simulink model "Simulador_Simulink"  (R2019b)
settings: Solver=FixedStepAuto  StartTime=0.0  StopTime=0.5  FixedStep=1e-6  RelTol=1e-3
model workspace (MAT data in the model file):
  SELDACA = 0
  SELPWM1A = 0
  SELPWM1B = 0
  SELPWM2A = 0
  SELPWM2B = 0
  SELPWM3A = 0
  SELPWM3B = 0
  Salidas_Reales = 0
values from neighbouring files (symbols this model uses):
  Dec = 1    [Sotfware_Matlab.m]
  Freq_Conmutacion = 10e3    (= 10000)    [Sotfware_Matlab.m]
  Ib = 2.5    [Sotfware_Matlab.m]
  Ireg_PI = tan((90 + Fc_pi)*pi/180)/wo_pi    [Sotfware_Matlab.m]
  Kreg_P = 1/AP    [Sotfware_Matlab.m]
  Kreg_PI = Ac_pi*Ireg_PI*wo_pi / sqrt(1 + (Ireg_PI*wo_pi)^2)    [Sotfware_Matlab.m]
  Lb = Zb/wb    [Sotfware_Matlab.m]
  Lpu = X_ind/ Lb    [Sotfware_Matlab.m]
  m = 0.5    [Sotfware_Matlab.m]
  Rpu = R_ind / Zb    [Sotfware_Matlab.m]
  T_pwm = 1/Freq_Conmutacion    (= 0.0001)    [Sotfware_Matlab.m]
  Ub = 0.61*Vdc / sqrt(3)    [Sotfware_Matlab.m]
  Vdc = 48    [Sotfware_Matlab.m]
  w1pu = 1    [Sotfware_Matlab.m]
  Zb = Ub/Ib    [Sotfware_Matlab.m]
libraries: powerlib x12, simulink x3, eeTransforms x3, electricdrivelib x1
settings Model: ParameterArgumentNames=SELDACA,SELPWM1A,SELPWM1B,SELPWM2A,SELPWM2B,SELPWM3A,SELPWM3B,Salidas_Reales  OrderedModelArguments=off  Creator=jorgesuarezporras  LastModifiedBy=jorge
settings SFSimCC: CustomCodeUndefinedFunction=UseInterfaceOnly

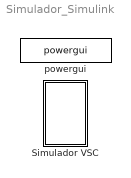
== system Simulador_Simulink ==
  Simulador VSC : Subsystem  mask{Parameter1A=Id, Parameter1B=Id Referencia, Parameter2A=Iq, Parameter2B=Iq Referencia, ParameterDAC=Ángulo transformada de Park, Parameter3A=Va, Parameter3B=Ia, Id_simulink=1, Iq_simulink=1, refd=Constante, refq=Constante, control=Control PI, K_proporcional=Kreg_P, b_proporcional=1, K_integral=Kreg_PI, I_integral=Ireg_PI, b_integral=1, tipolazo=Lazo Cerrado, mandod=0, mandoq=0, acoplamiento=on}
      mask prompts: Parameter1A "PWM1A"; Parameter1B "PWM1B"; Parameter2A "PWM2A"; Parameter2B "PWM2B"; ParameterDAC "DAC A"; Parameter3A "PWM3A"; Parameter3B "PWM3B"; Id_simulink "Id Referencia"; Iq_simulink "Iq Referencia"; refd "Forma de onda de referencia Id"; refq "Forma de onda de referencia Iq"; control "Selecciona el Control"; K_proporcional "K:"; b_proporcional "b:"; K_integral "K:"; I_integral "I:"; b_integral "b:"; tipolazo "Tipo de lazo"; mandod "Tensión de mando eje d  (md)"; mandoq "Tensión de mando eje q (mq)"
      mask init:
      | switch Parameter1A
      |     case 1
      |         SELPWM1A = 1;
      |     case 2
      |         SELPWM1A = 2;
      |     case 3
      |         SELPWM1A = 3;
      |     case 4
      |         SELPWM1A = 4;
      |     case 5
      |         SELPWM1A = 5;
      |     case 6
      |         SELPWM1A = 6;
      |     case 7
      |         SELPWM1A = 7;
      |     otherwise
      |         SELPWM1A = -1;
      | end
      | 
      | switch Parameter1B
      |     case 1
      |         SELPWM1B = 1;
      |     case 2
      |         SELPWM1B = 2;
      |     case 3
      |         SELPWM1B = 3;
      |     case 4
      |         SELPWM1B = 4;
      |     case 5
      |         SELPWM1B = 5;
      |     case 6
      |         SELPWM1B = 6;
      |     case 7
      |         SELPWM1B = 7;
      |     otherwise
      |         SELPWM1B = -1;
      | end
      | switch Parameter2A
      |     case 1
      |         SELPWM2A = 1;
      |     case 2
      |         SELPWM2A = 2;
      |     case 3
      |         SELPWM2A = 3;
      |     case 4
      |         SELPWM2A = 4;
      |     case 5
      |         SELPWM2A = 5;
      |     case 6
      |         SELPWM2A = 6;
      |     case 7
      |         SELPWM2A = 7;
      |     otherwise
      |         SELPWM2A = -1;
      | end
      | 
      | switch Parameter2B
      |     case 1
      |         SELPWM2B = 1;
      |     case 2
      |         SELPWM2B = 2;
      |     case 3
      |         SELPWM2B = 3;
      |     case 4
      |         SELPWM2B = 4;
      |     case 5
      |         SELPWM2B = 5;
      |     case 6
      |         SELPWM2B = 6;
      |     case 7
      |         SELPWM2B = 7;
      |     otherwise
      |         SELPWM2B = -1;
      | end
      | 
      | switch ParameterDAC
      |     case 1
      |         SELDACA = 1;
      |     case 2
      |         SELDACA = 2;
      |     case 3
      |         SELDACA = 3;
      |     case 4
      |         SELDACA = 4;
      |     case 5
      |         SELDACA = 5;
      |     case 6
      |         SELDACA = 6;
      |     case 7
      |         SELDACA = 7;
      |     otherwise
      |         SELDACA = -1;
      | end
      | switch Parameter3A
      |     case 1
      |         SELPWM3A = 8;
      |     case 2
      |         SELPWM3A = 9;
      |     case 3
      |         SELPWM3A = 10;
      |     case 4
      |         SELPWM3A = 11;
      |     case 5
      |         SELPWM3A = 12;
      |     case 6
      |         SELPWM3A = 13;
      |     otherwise
      |         SELPWM3A = -1;
      | end
      | switch Parameter3B
      |     case 1
      |         SELPWM3B = 8;
      |     case 2
      |         SELPWM3B = 9;
      |     case 3
      |         SELPWM3B = 10;
      |     case 4
      |         SELPWM3B = 11;
      |     case 5
      |         SELPWM3B = 12;
      |     case 6
      |         SELPWM3B = 13;
      |     otherwise
      |         SELPWM3B = -1;
      | end
      |        
      | switch refd
      |     case 1
      |         Id_ref_const = 1;
      |         Id_pulse = 0;
      |         Id_sin = 0;
      |     case 2
      |         Id_ref_const = 0;
      |         Id_pulse = 1;
      |         Id_sin = 0;        
      |     case 3
      |         Id_ref_const = 0;
      |         Id_pulse = 0;
      |         Id_sin = 1;
      | end
      | 
      | switch refq
      |     case 1
      |         Iq_ref_const = 1;
      |         Iq_pulse = 0;
      |         Iq_sin = 0;
      |     case 2
      |         Iq_ref_const = 0;
      |         Iq_pulse = 1;
      |         Iq_sin = 0;        
      |     case 3
      |         Iq_ref_const = 0;
      |         Iq_pulse = 0;
      |         Iq_sin = 1;
      | end
      | 
      | switch control
      |     case 1
      |         Control_P = 1;
      |         Control_PI = 0;
      |         I_integral = 1;
      |     case 2
      |         Control_P = 0;
      |         Control_PI = 1;
      | end
      | 
      | switch tipolazo
      |     case 1
      |         open = 0;
      |         a_d = mandod;
      |         a_q = mandoq;
      |     case 2
      |         open = 1;
      |         a_d = 0;
      |         a_q = 0;
      | end
      | 
      | if acoplamiento == 1
      |         open_Id = 1;
      |         open_Iq = 1;
      | else 
      |     open_Id = 0;
      |     open_Iq = 0;
      | end
      | % 
      | % if reales == 1
      | %         Salidas_Reales = 1;
      | % else 
      | %     Salidas_Reales = 0;
      | % end
      mask TypeOptions Parameter1A: Id | Iq | Id Referencia | Iq Referencia | md | mq | Ángulo transformada de Park
      mask TypeOptions Parameter1B: Id | Iq | Id Referencia | Iq Referencia | md | mq | Ángulo transformada de Park
      mask TypeOptions Parameter2A: Id | Iq | Id Referencia | Iq Referencia | md | mq | Ángulo transformada de Park
      mask TypeOptions Parameter2B: Id | Iq | Id Referencia | Iq Referencia | md | mq | Ángulo transformada de Park
      mask TypeOptions ParameterDAC: Id | Iq | Id Referencia | Iq Referencia | md | mq | Ángulo transformada de Park
      mask TypeOptions Parameter3A: Va | Vb | Vc | Ia | Ib | Ic
      mask TypeOptions Parameter3B: Va | Vb | Vc | Ia | Ib | Ic
      mask TypeOptions refd: Constante | Pulsos | Senoidal
      mask TypeOptions refq: Constante | Pulsos | Senoidal
      mask TypeOptions control: Control P | Control PI
      mask TypeOptions tipolazo: Lazo Abierto | Lazo Cerrado
      mask DialogControl Container7 Prompt: Salidas
      mask DialogControl Container9 Prompt: Referencias
      mask DialogControl Container12 Prompt: Controles
      mask DialogControl Container22 Prompt: Control Proporcional
      mask DialogControl Container24 Prompt: Control Proporcional - Integral
      mask DialogControl Container19 Prompt: Lazo
      mask DialogControl Container17 Prompt: Lazo Abierto
      mask DialogControl Container18 Prompt: Acoplamiento / Desacoplamiento
      mask Display: image('click.png'); % Use "Edit Image" on toolstrip to change.
  powergui : powerlib/powergui  Priority=1  SimulationMode=Continuous  SampleTime=50e-6  frequency=60  Iterations=50  frequencyindice=0  Pbase=100e6  ErrMax=1e-4  UnitsV=kV  UnitsW=MW  buscounter=0  FunctionMessages=off  echomessages=off  EnableUseOfTLC=off  CurrentSourceSwitches=off  DisableSnubberDevices=off  DisableRonSwitches=off  DisableVfSwitches=off  DisplayEquations=off  AutomaticDiscreteSolvers=off  SolverType=Tustin/Backward Euler (TBE)  Interpol=off  ExternalGateDelay=off  methode=off  Ts=100  x0status=blocks  SPID=on  SwTol=0  HookPort=off  NonlinearTolerance=0  nMaxIteration=15  ContinueOnMaxIteration=off  RestoreLinks=warning  ResistiveCurrentMeasurement=off  Frange=[0:2:500]  Ylog=off  Xlog=on  ShowGrid=off  save=off  variable=ZData  structure=0  ZoomFFT=off  StartTime=0.0  cycles=1  DisplayStyle=1  fundamental=60  FreqAxis=off  MaxFrequency=1000  frequencyindicesteady=1  RmsSteady=1  display=off
      settings: SourceProductName=Simscape Electrical

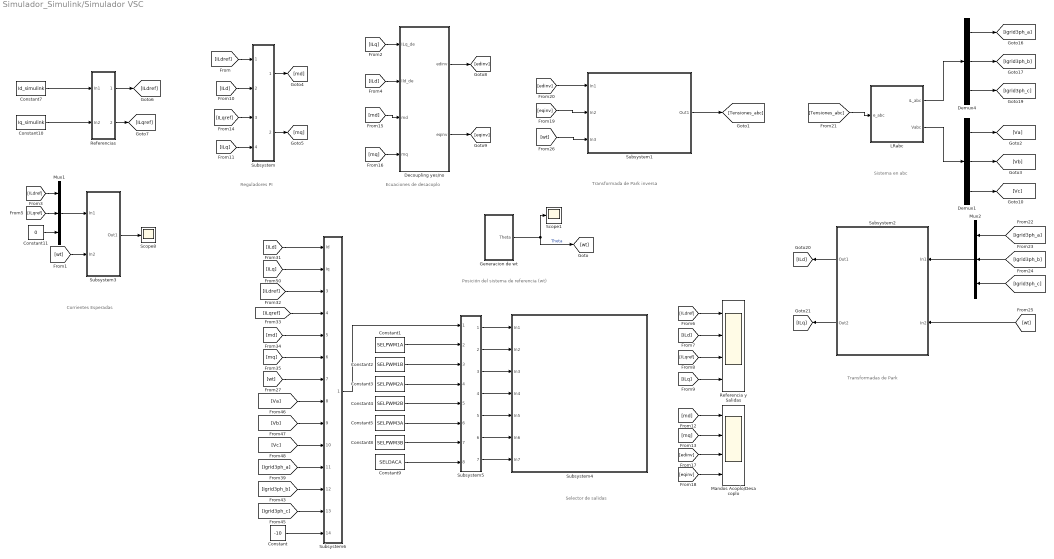
== system Simulador_Simulink/Simulador VSC ==
  note: Posición del sistema de referencia (wt)
  note: Transformadas de Park
  note: Transformada de Park inversa
  note: Ecuaciones de desacoplo
  note: Reguladores PI
  note: Sistema en abc
  note: Corrientes Esperadas
  note: Selector de salidas
  Constant : Constant  Value=-10
  Constant1 : Constant  Value=SELPWM1A  SampleTime=-1
  Constant10 : Constant  Value=Iq_simulink  SampleTime=-1
  Constant11 : Constant  Value=0
  Constant2 : Constant  Value=SELPWM1B  SampleTime=-1
  Constant3 : Constant  Value=SELPWM2A  SampleTime=-1
  Constant4 : Constant  Value=SELPWM2B  SampleTime=-1
  Constant5 : Constant  Value=SELPWM3A
  Constant7 : Constant  Value=Id_simulink  SampleTime=-1
  Constant8 : Constant  Value=SELPWM3B  SampleTime=-1
  Constant9 : Constant  Value=SELDACA  SampleTime=-1
  Decoupling yes/no : Subsystem
  Demux1 : Demux  Outputs=3
  Demux4 : Demux  Outputs=3
  Generacion de wt : Subsystem
  LRabc : Subsystem
  Mandos Acoplo/Desacoplo : Scope  NumInputPorts=4
  Mux1 : Mux  Inputs=3
  Mux2 : Mux  Inputs=3
  Referencia y Salidas : Scope  NumInputPorts=4
  Referencias : Subsystem
  Scope1 : Scope
  Scope8 : Scope
  Subsystem : Subsystem
  Subsystem1 : Subsystem
  Subsystem2 : Subsystem
  Subsystem3 : Subsystem
  Subsystem4 : Subsystem
  Subsystem5 : Subsystem
  Subsystem6 : Subsystem
  wires:
  [Igrid3ph_a] -> Mux2/1
  [eqinv] -> Mandos Acoplo/Desacoplo/4
  [md] -> Mandos Acoplo/Desacoplo/1
  Constant11/1 -> Mux1/3
  [ILqref] -> Referencia y Salidas/3
  [edinv] -> Mandos Acoplo/Desacoplo/3
  Decoupling yes/no/1(edinv) -> [edinv]
  [ILqref] -> Mux1/2
  [ILdref] -> Referencia y Salidas/1
  [ILd] -> Referencia y Salidas/2
  [ILq] -> Decoupling yes/no/1(ILq_de)
  [ILdref] -> Mux1/1
  [Igrid3ph_b] -> Mux2/2
  [ILd] -> Decoupling yes/no/2(Ild_de)
  [mq] -> Mandos Acoplo/Desacoplo/2
  [ILq] -> Referencia y Salidas/4
  [Igrid3ph_c] -> Mux2/3
  Decoupling yes/no/2(eqinv) -> [eqinv]
  Mux2/1 -> Subsystem2/1(In1)
  Generacion de wt/1(Theta) -> [wt], Scope1/1  "Theta"
  Referencias/1(Out1) -> [ILdref]
  Constant7/1 -> Referencias/1(In1)
  Constant10/1 -> Referencias/2(In2)
  Referencias/2(Out2) -> [ILqref]
  Subsystem/2(Out2) -> [mq]
  Subsystem/1(Out1) -> [md]
  [ILdref] -> Subsystem/1(In1)
  [ILd] -> Subsystem/2(In2)
  [ILqref] -> Subsystem/3(In3)
  [ILq] -> Subsystem/4(In4)
  [md] -> Decoupling yes/no/3(md)
  [mq] -> Decoupling yes/no/4(mq)
  Demux4/1 -> [Igrid3ph_a]
  Demux4/2 -> [Igrid3ph_b]
  Demux4/3 -> [Igrid3ph_c]
  [wt] -> Subsystem2/2(In2)
  Subsystem2/1(Out1) -> [ILd]
  Subsystem2/2(Out2) -> [ILq]
  LRabc/1(iL_abc) -> Demux4/1
  [edinv] -> Subsystem1/1(In1)
  [eqinv] -> Subsystem1/2(In2)
  [wt] -> Subsystem1/3(In3)
  Subsystem1/1(Out1) -> [Tensiones_abc]
  [Tensiones_abc] -> LRabc/1(e_abc)
  Mux1/1 -> Subsystem3/1(In1)
  [wt] -> Subsystem3/2(In2)
  Subsystem3/1(Out1) -> Scope8/1
  Constant9/1 -> Subsystem5/8(In8)
  Constant1/1 -> Subsystem5/2(In2)
  Constant3/1 -> Subsystem5/4(In4)
  Constant5/1 -> Subsystem5/6(In6)
  Constant4/1 -> Subsystem5/5(In5)
  Constant2/1 -> Subsystem5/3(In3)
  Constant8/1 -> Subsystem5/7(In7)
  Demux1/3 -> [Vc]
  Demux1/2 -> [Vb]
  Demux1/1 -> [Va]
  LRabc/2(Vabc) -> Demux1/1
  [ILd] -> Subsystem6/1(Id)
  [ILq] -> Subsystem6/2(Iq)
  [ILdref] -> Subsystem6/3(In3)
  [ILqref] -> Subsystem6/4(In4)
  [md] -> Subsystem6/5(In5)
  [mq] -> Subsystem6/6(In6)
  [wt] -> Subsystem6/7(In7)
  [Va] -> Subsystem6/8(In8)
  [Vb] -> Subsystem6/9(In9)
  [Vc] -> Subsystem6/10(In10)
  [Igrid3ph_a] -> Subsystem6/11(In11)
  [Igrid3ph_b] -> Subsystem6/12(In12)
  [Igrid3ph_c] -> Subsystem6/13(In13)
  Constant/1 -> Subsystem6/14(In1)
  Subsystem6/1(Out1) -> Subsystem5/1(In1)
  Subsystem5/1(Out7) -> Subsystem4/1(In1)
  Subsystem5/2(Out1) -> Subsystem4/2(In2)
  Subsystem5/3(Out2) -> Subsystem4/3(In3)
  Subsystem5/4(Out3) -> Subsystem4/4(In4)
  Subsystem5/5(Out4) -> Subsystem4/5(In5)
  Subsystem5/6(Out5) -> Subsystem4/6(In6)
  Subsystem5/7(Out6) -> Subsystem4/7(In7)

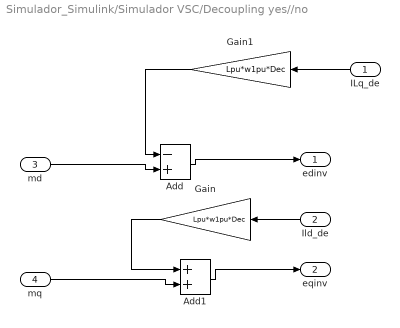
== system Simulador_Simulink/Simulador VSC/Decoupling yes//no ==
  ILq_de : Inport
  Ild_de : Inport  Port=2
  md : Inport  Port=3
  mq : Inport  Port=4
  Add : Sum  Inputs=-+
  Add1 : Sum
  Gain : Gain  Gain=Lpu*w1pu*Dec
  Gain1 : Gain  Gain=Lpu*w1pu*Dec
  edinv : Outport  VectorParamsAs1DForOutWhenUnconnected=off
  eqinv : Outport  Port=2  VectorParamsAs1DForOutWhenUnconnected=off
  wires:
  Add1/1 -> eqinv/1
  ILq_de/1 -> Gain1/1
  mq/1 -> Add1/2
  Gain1/1 -> Add/1
  Ild_de/1 -> Gain/1
  Gain/1 -> Add1/1
  Add/1 -> edinv/1
  md/1 -> Add/2

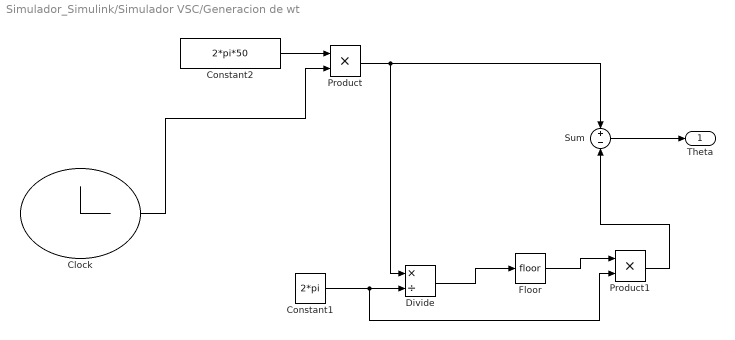
== system Simulador_Simulink/Simulador VSC/Generacion de wt ==
  Clock : Clock
  Constant1 : Constant  Value=2*pi
  Constant2 : Constant  Value=2*pi*50
  Divide : Product  Inputs=*/
  Floor : Rounding
  Product : Product
  Product1 : Product
  Sum : Sum  Inputs=+-
  Theta : Outport  VectorParamsAs1DForOutWhenUnconnected=off
  wires:
  Product/1 -> Sum/1, Divide/1
  Constant1/1 -> Divide/2, Product1/2
  Product1/1 -> Sum/2
  Sum/1 -> Theta/1
  Divide/1 -> Floor/1
  Floor/1 -> Product1/1
  Constant2/1 -> Product/1
  Clock/1 -> Product/2

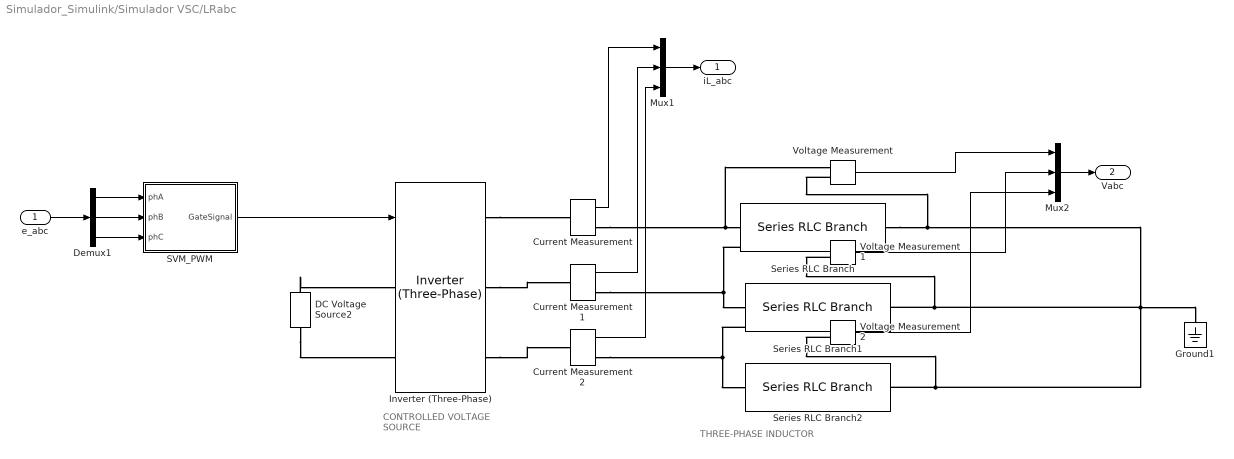
== system Simulador_Simulink/Simulador VSC/LRabc ==
  note: CONTROLLED VOLTAGE
      | SOURCE
  note: THREE-PHASE INDUCTOR
  e_abc : Inport
  Current Measurement : powerlib/Measurements/Current Measurement  PhasorSimulation=off  OutputType=Complex  PSBequivalent=0
      settings: SourceProductName=Simscape Electrical
  Current Measurement1 : powerlib/Measurements/Current Measurement  PhasorSimulation=off  OutputType=Complex  PSBequivalent=0
      settings: SourceProductName=Simscape Electrical
  Current Measurement2 : powerlib/Measurements/Current Measurement  PhasorSimulation=off  OutputType=Complex  PSBequivalent=0
      settings: SourceProductName=Simscape Electrical
  DC Voltage Source2 : powerlib/Electrical Sources/DC Voltage Source  Amplitude=Vdc  Measurements=None
      settings: SourceProductName=Simscape Electrical
  Demux1 : Demux  Outputs=3
  Ground1 : powerlib/Elements/Ground  LConnTagsString=a
      settings: SourceProductName=Simscape Electrical
  Inverter (Three-Phase) : electricdrivelib/Fundamental Drive Blocks/Inverter (Three-Phase)  LabelModeActiveChoice=Detailed  detailLevel=Detailed  driveType=Field-oriented control  Ts=2e-6  SnubberResistance=10e3  SnubberCapacitance=inf  Device=IGBT / Diodes  Ron=1e-3  ForwardVoltages=[1.2,1.2]  GTOparameters=[1e-6,2e-6]  IGBTparameters=[1e-6,2e-6]  Measurements=All voltages and currents  converterType=Inverter  SourceFrequency=60  ReferenceFrame=Rotor  dqInductances=[8.5e-3,8.5e-3]  Inductance=8.5e-3  Ls=0  Resistance=0.2  Flux=0.175  Stator_sm=[2.01e-3,4.289e-4,4.477e-3,1.354e-3]  Stator_im=[14.85e-3,0.3027e-3]  Rotor=[9.295e-3,0.3027e-3]  Lm=10.46e-3  p=4
      settings: AttributesFormatString=%<BlockChoice>  SourceProductName=Simscape Electrical  SourceProductBaseCode=PS
  Mux1 : Mux  Inputs=3
  Mux2 : Mux  Inputs=3
  SVM_PWM : Subsystem
  Series RLC Branch : powerlib/Elements/Series RLC Branch  LConnTagsString=__new0  RConnTagsString=__new0  BranchType=RL  Resistance=Rpu*Zb  Inductance=Lpu*Lb  SetiL0=off  InitialCurrent=0  Capacitance=1e-6  Setx0=off  InitialVoltage=0  Measurements=Branch current
      settings: SourceProductName=Simscape Electrical
  Series RLC Branch1 : powerlib/Elements/Series RLC Branch  LConnTagsString=__new0  RConnTagsString=__new0  BranchType=RL  Resistance=Rpu*Zb  Inductance=Lpu*Lb  SetiL0=off  InitialCurrent=0  Capacitance=1e-6  Setx0=off  InitialVoltage=0  Measurements=Branch current
      settings: SourceProductName=Simscape Electrical
  Series RLC Branch2 : powerlib/Elements/Series RLC Branch  LConnTagsString=__new0  RConnTagsString=__new0  BranchType=RL  Resistance=Rpu*Zb  Inductance=Lpu*Lb  SetiL0=off  InitialCurrent=0  Capacitance=1e-6  Setx0=off  InitialVoltage=0  Measurements=Branch current
      settings: SourceProductName=Simscape Electrical
  Voltage Measurement : powerlib/Measurements/Voltage Measurement  PhasorSimulation=off  OutputType=Complex  PSBequivalent=0
      settings: SourceProductName=Simscape Electrical
  Voltage Measurement1 : powerlib/Measurements/Voltage Measurement  PhasorSimulation=off  OutputType=Complex  PSBequivalent=0
      settings: SourceProductName=Simscape Electrical
  Voltage Measurement2 : powerlib/Measurements/Voltage Measurement  PhasorSimulation=off  OutputType=Complex  PSBequivalent=0
      settings: SourceProductName=Simscape Electrical
  iL_abc : Outport  VectorParamsAs1DForOutWhenUnconnected=off
  Vabc : Outport  Port=2  VectorParamsAs1DForOutWhenUnconnected=off
  wires:
  Current Measurement1/1 -> Mux1/2
  Current Measurement2/1 -> Mux1/3
  Current Measurement/1 -> Mux1/1
  Mux1/1 -> iL_abc/1
  Demux1/1 -> SVM_PWM/1(phA)
  Demux1/3 -> SVM_PWM/3(phC)
  SVM_PWM/1(GateSignal) -> Inverter (Three-Phase)/1
  Demux1/2 -> SVM_PWM/2(phB)
  e_abc/1 -> Demux1/1
  Voltage Measurement/1 -> Mux2/1
  Voltage Measurement1/1 -> Mux2/2
  Voltage Measurement2/1 -> Mux2/3
  Mux2/1 -> Vabc/1
  connections:
  Voltage Measurement/LConn2 -- Series RLC Branch/RConn1 -- Voltage Measurement1/LConn2 -- Series RLC Branch1/RConn1 -- Ground1/LConn1 -- Voltage Measurement2/LConn2 -- Series RLC Branch2/RConn1
  Current Measurement1/RConn1 -- Series RLC Branch1/LConn1 -- Voltage Measurement1/LConn1
  Inverter (Three-Phase)/RConn2 -- Current Measurement1/LConn1
  Current Measurement/RConn1 -- Voltage Measurement/LConn1 -- Series RLC Branch/LConn1
  Inverter (Three-Phase)/RConn1 -- Current Measurement/LConn1
  Inverter (Three-Phase)/RConn3 -- Current Measurement2/LConn1
  Current Measurement2/RConn1 -- Series RLC Branch2/LConn1 -- Voltage Measurement2/LConn1
  DC Voltage Source2/RConn1 -- Inverter (Three-Phase)/LConn1
  DC Voltage Source2/LConn1 -- Inverter (Three-Phase)/LConn2

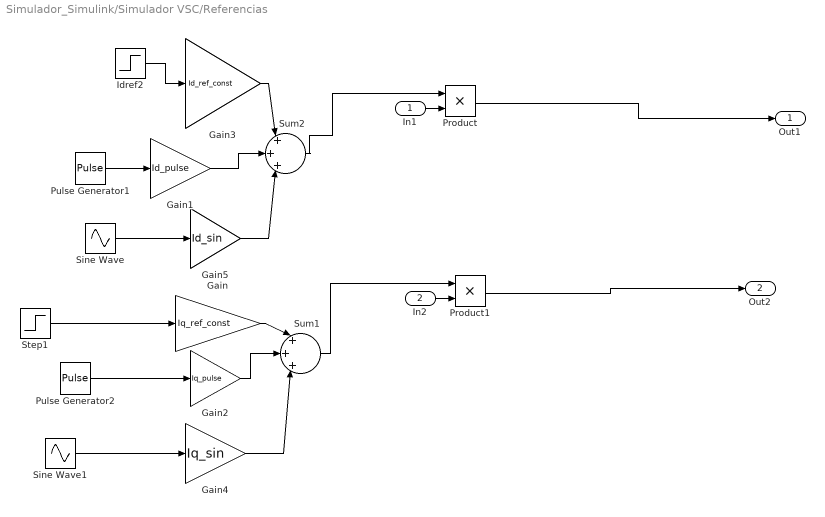
== system Simulador_Simulink/Simulador VSC/Referencias ==
  In1 : Inport
  In2 : Inport  Port=2
  Gain : Gain  Gain=Iq_ref_const
  Gain1 : Gain  Gain=Id_pulse
  Gain2 : Gain  Gain=Iq_pulse
  Gain3 : Gain  Gain=Id_ref_const
  Gain4 : Gain  Gain=Iq_sin
  Gain5 : Gain  Gain=Id_sin
  Idref2 : Step  Time=0.05
  Product : Product
  Product1 : Product
  Pulse Generator1 : DiscretePulseGenerator  Period=100000  PulseWidth=100000*0.5  SampleTime=T_pwm  VectorParams1D=off
  Pulse Generator2 : DiscretePulseGenerator  Period=100000  PulseWidth=100000*0.5  PhaseDelay=100000*0.3  SampleTime=T_pwm  VectorParams1D=off
  Sine Wave : Sin  SineType=Sample based  Samples=10000  SampleTime=T_pwm
  Sine Wave1 : Sin  SineType=Sample based  Samples=10000  SampleTime=T_pwm
  Step1 : Step  Time=0.25
  Sum1 : Sum  Inputs=|+|+|+|
  Sum2 : Sum  Inputs=|+|+|+|
  Out1 : Outport  VectorParamsAs1DForOutWhenUnconnected=off
  Out2 : Outport  Port=2  VectorParamsAs1DForOutWhenUnconnected=off
  wires:
  In2/1 -> Product1/2
  In1/1 -> Product/2
  Product1/1 -> Out2/1
  Product/1 -> Out1/1
  Idref2/1 -> Gain3/1
  Pulse Generator1/1 -> Gain1/1
  Sum2/1 -> Product/1
  Sum1/1 -> Product1/1
  Pulse Generator2/1 -> Gain2/1
  Step1/1 -> Gain/1
  Gain/1 -> Sum1/1
  Gain3/1 -> Sum2/1
  Gain2/1 -> Sum1/2
  Gain1/1 -> Sum2/2
  Sine Wave/1 -> Gain5/1
  Sine Wave1/1 -> Gain4/1
  Gain4/1 -> Sum1/3
  Gain5/1 -> Sum2/3

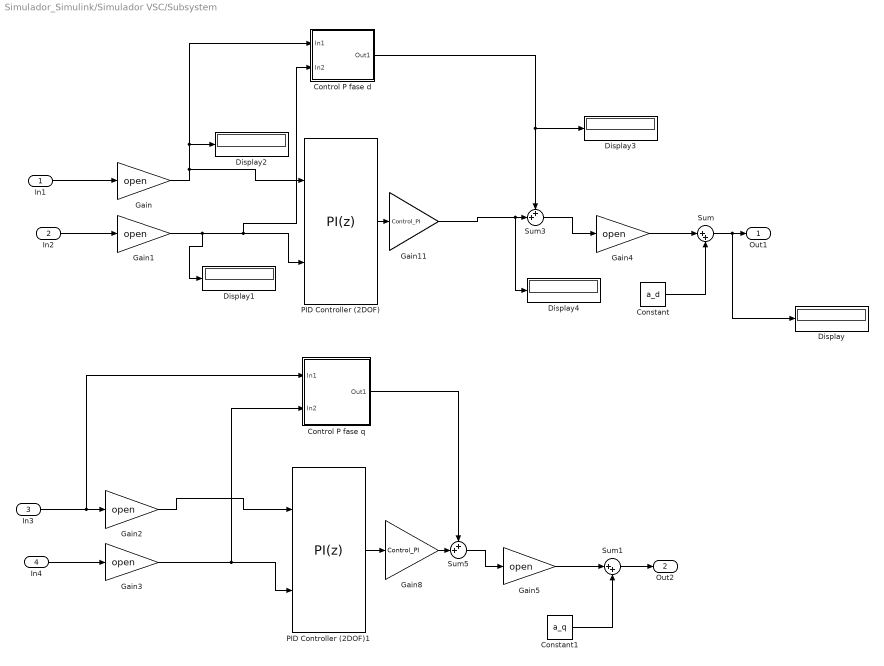
== system Simulador_Simulink/Simulador VSC/Subsystem ==
  In1 : Inport
  In2 : Inport  Port=2
  In3 : Inport  Port=3
  In4 : Inport  Port=4
  Constant : Constant  Value=a_d
  Constant1 : Constant  Value=a_q
  Control P fase d : Subsystem
  Control P fase q : Subsystem
  Display{,1..4} (5 alike) : Display
  Gain{,1..5} (6 alike) : Gain  Gain=open
  Gain11 : Gain  Gain=Control_PI
  Gain8 : Gain  Gain=Control_PI
  PID Controller (2DOF) : simulink/Continuous/PID Controller (2DOF)  Controller=PI  Form=Ideal  TimeDomain=Discrete-time  SampleTime=-1  IntegratorMethod=Forward Euler  FilterMethod=Forward Euler  ControllerParametersSource=internal  P=K_integral  I=K_integral/I_integral  D=0  UseFilter=on  N=100  b=b_integral  c=1  TunerSelectOption=Frequency Response Based  InitialConditionSource=internal  InitialConditionForIntegrator=0  InitialConditionForFilter=0  DifferentiatorICPrevScaledInput=0  ExternalReset=none  TrackingMode=off  Kt=1  LimitOutput=off  UpperSaturationLimit=1.5  LowerSaturationLimit=-3  LinearizeAsGain=on  AntiWindupMode=none  Kb=1  POutMin=[]  POutMax=[]  IOutMin=[]  IOutMax=[]  DOutMin=[]  DOutMax=[]  NOutMin=[]  NOutMax=[]  bOutMin=[]  bOutMax=[]  cOutMin=[]  cOutMax=[]  SumOutMin=[]  SumOutMax=[]  SaturationOutMin=[]  SaturationOutMax=[]  PParamMin=[]  PParamMax=[]  IParamMin=[]  IParamMax=[]  DParamMin=[]  DParamMax=[]  NParamMin=[]  NParamMax=[]  bParamMin=[]  bParamMax=[]  cParamMin=[]  cParamMax=[]  KbParamMin=[]  KbParamMax=[]  KtParamMin=[]  KtParamMax=[]  KbOutMin=[]  KbOutMax=[]  KtOutMin=[]  KtOutMax=[]  IntegratorOutMin=[]  IntegratorOutMax=[]  FilterOutMin=[]  FilterOutMax=[]  SumI1OutMin=[]  SumI1OutMax=[]  SumI2OutMin=[]  SumI2OutMax=[]  SumI3OutMin=[]  SumI3OutMax=[]  SumI4OutMin=[]  SumI4OutMax=[]  SumDOutMin=[]  SumDOutMax=[]  Sum1OutMin=[]  Sum1OutMax=[]  Sum2OutMin=[]  Sum2OutMax=[]  Sum3OutMin=[]  Sum3OutMax=[]  DifferentiatorOutMin=[]  DifferentiatorOutMax=[]  FilterDiffOutCoefMin=[]  FilterDiffOutCoefMax=[]  ReciprocalOutMin=[]  ReciprocalOutMax=[]  SumDenOutMin=[]  SumDenOutMax=[]  SumNumOutMin=[]  SumNumOutMax=[]  DivideOutMin=[]  DivideOutMax=[]  IntegratorContinuousStateAttributes=''  IntegratorStateMustResolveToSignalObject=off  IntegratorRTWStateStorageClass=Auto  FilterContinuousStateAttributes=''  FilterStateMustResolveToSignalObject=off  FilterRTWStateStorageClass=Auto  ParallelPVariant=Passthrough  IdealPVariant=InternalParameters  IVariant=InternalParameters  DVariant=Disabled  bVariant=InternalParameters  cVariant=Disabled  IntegratorVariant=Discrete  SatVariant=Disabled  AWVariant=Passthrough  PCopyVariant=Disabled  TRVariant=Disabled  FdbkBlocksVariant=Forward  IdealPFdbkVariant=Disabled  SatFdbkVariant=Disabled  DerivativeFilterVariant=Disabled  NVariant=Disabled  NCopyVariant=Disabled_SignalSpec  FilterICVariant=Disabled  IntegratorICVariant=InternalICs  ExternalResetVariant=Disabled  TRSumVariant=Passthrough  SumFdbkVariant=Disabled  SumVariant=Sum_PI
  PID Controller (2DOF)1 : simulink/Continuous/PID Controller (2DOF)  Controller=PI  Form=Ideal  TimeDomain=Discrete-time  SampleTime=-1  IntegratorMethod=Forward Euler  FilterMethod=Forward Euler  ControllerParametersSource=internal  P=K_integral  I=K_integral/I_integral  D=0  UseFilter=on  N=100  b=b_integral  c=1  TunerSelectOption=Frequency Response Based  InitialConditionSource=internal  InitialConditionForIntegrator=0  InitialConditionForFilter=0  DifferentiatorICPrevScaledInput=0  ExternalReset=none  TrackingMode=off  Kt=1  LimitOutput=off  UpperSaturationLimit=1.5  LowerSaturationLimit=-3  LinearizeAsGain=on  AntiWindupMode=none  Kb=1  POutMin=[]  POutMax=[]  IOutMin=[]  IOutMax=[]  DOutMin=[]  DOutMax=[]  NOutMin=[]  NOutMax=[]  bOutMin=[]  bOutMax=[]  cOutMin=[]  cOutMax=[]  SumOutMin=[]  SumOutMax=[]  SaturationOutMin=[]  SaturationOutMax=[]  PParamMin=[]  PParamMax=[]  IParamMin=[]  IParamMax=[]  DParamMin=[]  DParamMax=[]  NParamMin=[]  NParamMax=[]  bParamMin=[]  bParamMax=[]  cParamMin=[]  cParamMax=[]  KbParamMin=[]  KbParamMax=[]  KtParamMin=[]  KtParamMax=[]  KbOutMin=[]  KbOutMax=[]  KtOutMin=[]  KtOutMax=[]  IntegratorOutMin=[]  IntegratorOutMax=[]  FilterOutMin=[]  FilterOutMax=[]  SumI1OutMin=[]  SumI1OutMax=[]  SumI2OutMin=[]  SumI2OutMax=[]  SumI3OutMin=[]  SumI3OutMax=[]  SumI4OutMin=[]  SumI4OutMax=[]  SumDOutMin=[]  SumDOutMax=[]  Sum1OutMin=[]  Sum1OutMax=[]  Sum2OutMin=[]  Sum2OutMax=[]  Sum3OutMin=[]  Sum3OutMax=[]  DifferentiatorOutMin=[]  DifferentiatorOutMax=[]  FilterDiffOutCoefMin=[]  FilterDiffOutCoefMax=[]  ReciprocalOutMin=[]  ReciprocalOutMax=[]  SumDenOutMin=[]  SumDenOutMax=[]  SumNumOutMin=[]  SumNumOutMax=[]  DivideOutMin=[]  DivideOutMax=[]  IntegratorContinuousStateAttributes=''  IntegratorStateMustResolveToSignalObject=off  IntegratorRTWStateStorageClass=Auto  FilterContinuousStateAttributes=''  FilterStateMustResolveToSignalObject=off  FilterRTWStateStorageClass=Auto  ParallelPVariant=Passthrough  IdealPVariant=InternalParameters  IVariant=InternalParameters  DVariant=Disabled  bVariant=InternalParameters  cVariant=Disabled  IntegratorVariant=Discrete  SatVariant=Disabled  AWVariant=Passthrough  PCopyVariant=Disabled  TRVariant=Disabled  FdbkBlocksVariant=Forward  IdealPFdbkVariant=Disabled  SatFdbkVariant=Disabled  DerivativeFilterVariant=Disabled  NVariant=Disabled  NCopyVariant=Disabled_SignalSpec  FilterICVariant=Disabled  IntegratorICVariant=InternalICs  ExternalResetVariant=Disabled  TRSumVariant=Passthrough  SumFdbkVariant=Disabled  SumVariant=Sum_PI
  Sum : Sum  Inputs=|++
  Sum1 : Sum  Inputs=|++
  Sum3 : Sum  Inputs=++|
  Sum5 : Sum  Inputs=++|
  Out1 : Outport  VectorParamsAs1DForOutWhenUnconnected=off
  Out2 : Outport  Port=2  VectorParamsAs1DForOutWhenUnconnected=off
  wires:
  Gain4/1 -> Sum/1
  In3/1 -> Control P fase q/1(In1), Gain2/1
  PID Controller (2DOF)/1 -> Gain11/1
  Constant/1 -> Sum/2
  Gain3/1 -> Control P fase q/2(In2), PID Controller (2DOF)1/2
  In2/1 -> Gain1/1
  Gain/1 -> Control P fase d/1(In1), Display2/1, PID Controller (2DOF)/1
  Gain1/1 -> Display1/1, Control P fase d/2(In2), PID Controller (2DOF)/2
  PID Controller (2DOF)1/1 -> Gain8/1
  Sum/1 -> Display/1, Out1/1
  In4/1 -> Gain3/1
  Gain8/1 -> Sum5/2
  Gain2/1 -> PID Controller (2DOF)1/1
  In1/1 -> Gain/1
  Sum1/1 -> Out2/1
  Gain11/1 -> Display4/1, Sum3/2
  Sum5/1 -> Gain5/1
  Constant1/1 -> Sum1/2
  Gain5/1 -> Sum1/1
  Sum3/1 -> Gain4/1
  Control P fase q/1(Out1) -> Sum5/1
  Control P fase d/1(Out1) -> Display3/1, Sum3/1

== system Simulador_Simulink/Simulador VSC/Subsystem1 ==
  In1 : Inport
  In2 : Inport  Port=2
  In3 : Inport  Port=3
  Constant : Constant  Value=0
  Constant12 : Constant  Value=Ub
  Inverse Park Transform : eeTransforms/Inverse Park Transform  AxisAlignment=Q-axis  PowerInvariant=on
      settings: SourceProductName=Simscape Electrical
  Mux4 : Mux  Inputs=3
  Product : Product
  Out1 : Outport  VectorParamsAs1DForOutWhenUnconnected=off
  wires:
  Constant12/1 -> Product/2
  Constant/1 -> Mux4/3
  Inverse Park Transform/1 -> Product/1
  Product/1 -> Out1/1
  In2/1 -> Mux4/2
  In1/1 -> Mux4/1
  In3/1 -> Inverse Park Transform/2
  Mux4/1 -> Inverse Park Transform/1

== system Simulador_Simulink/Simulador VSC/Subsystem2 ==
  In1 : Inport
  In2 : Inport  Port=2
  Constant6 : Constant  Value=Ib
  Demux1 : Demux  Outputs=3
  Divide : Product  Inputs=*/
  Park Transform : eeTransforms/Park Transform  AxisAlignment=Q-axis  PowerInvariant=on
      settings: SourceProductName=Simscape Electrical
  Terminator1 : Terminator
  Out1 : Outport  VectorParamsAs1DForOutWhenUnconnected=off
  Out2 : Outport  Port=2  VectorParamsAs1DForOutWhenUnconnected=off
  wires:
  In1/1 -> Divide/1
  Demux1/2 -> Out2/1
  Divide/1 -> Park Transform/1
  Demux1/1 -> Out1/1
  In2/1 -> Park Transform/2
  Demux1/3 -> Terminator1/1
  Constant6/1 -> Divide/2
  Park Transform/1 -> Demux1/1

== system Simulador_Simulink/Simulador VSC/Subsystem3 ==
  In1 : Inport
  In2 : Inport  Port=2
  Gain : Gain  Gain=Ib
  Inverse Park Transform1 : eeTransforms/Inverse Park Transform  AxisAlignment=Q-axis  PowerInvariant=on
      settings: SourceProductName=Simscape Electrical
  Out1 : Outport  VectorParamsAs1DForOutWhenUnconnected=off
  wires:
  In1/1 -> Inverse Park Transform1/1
  Gain/1 -> Out1/1
  In2/1 -> Inverse Park Transform1/2
  Inverse Park Transform1/1 -> Gain/1

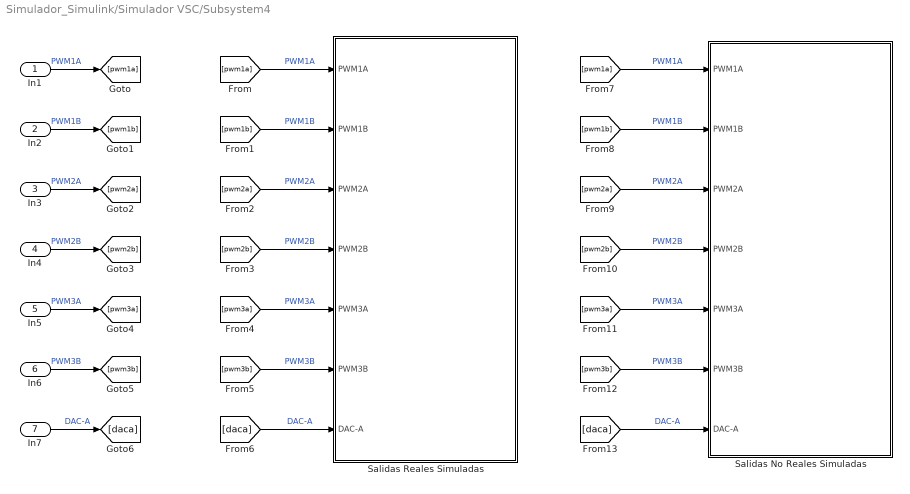
== system Simulador_Simulink/Simulador VSC/Subsystem4 ==
  In1 : Inport
  In2 : Inport  Port=2
  In3 : Inport  Port=3
  In4 : Inport  Port=4
  In5 : Inport  Port=5
  In6 : Inport  Port=6
  In7 : Inport  Port=7
  Salidas No Reales Simuladas : Subsystem
  Salidas Reales Simuladas : Subsystem
  wires:
  [pwm1a] -> Salidas Reales Simuladas/1(PWM1A)  "PWM1A"
  [pwm1b] -> Salidas Reales Simuladas/2(PWM1B)  "PWM1B"
  [pwm2a] -> Salidas Reales Simuladas/3(PWM2A)  "PWM2A"
  [pwm2b] -> Salidas Reales Simuladas/4(PWM2B)  "PWM2B"
  [pwm3a] -> Salidas Reales Simuladas/5(PWM3A)  "PWM3A"
  [pwm3b] -> Salidas Reales Simuladas/6(PWM3B)  "PWM3B"
  [daca] -> Salidas Reales Simuladas/7(DAC-A)  "DAC-A"
  [daca] -> Salidas No Reales Simuladas/7(DAC-A)  "DAC-A"
  [pwm3b] -> Salidas No Reales Simuladas/6(PWM3B)  "PWM3B"
  [pwm3a] -> Salidas No Reales Simuladas/5(PWM3A)  "PWM3A"
  [pwm2b] -> Salidas No Reales Simuladas/4(PWM2B)  "PWM2B"
  [pwm2a] -> Salidas No Reales Simuladas/3(PWM2A)  "PWM2A"
  [pwm1b] -> Salidas No Reales Simuladas/2(PWM1B)  "PWM1B"
  [pwm1a] -> Salidas No Reales Simuladas/1(PWM1A)  "PWM1A"
  In1/1 -> [pwm1a]  "PWM1A"
  In2/1 -> [pwm1b]  "PWM1B"
  In3/1 -> [pwm2a]  "PWM2A"
  In4/1 -> [pwm2b]  "PWM2B"
  In5/1 -> [pwm3a]  "PWM3A"
  In6/1 -> [pwm3b]  "PWM3B"
  In7/1 -> [daca]  "DAC-A"

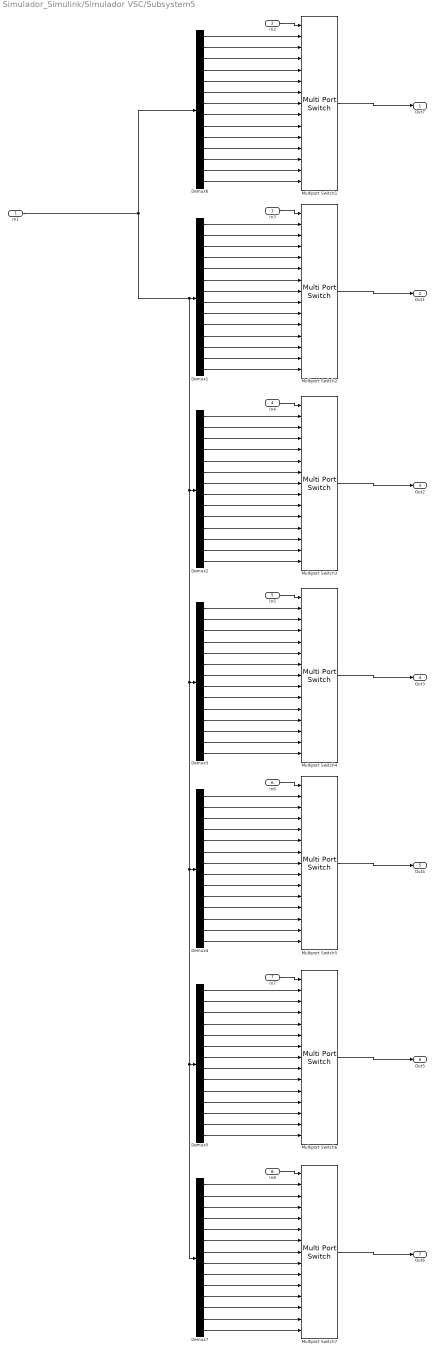
== system Simulador_Simulink/Simulador VSC/Subsystem5 ==
  In1 : Inport
  In2 : Inport  Port=2
  In3 : Inport  Port=3
  In4 : Inport  Port=4
  In5 : Inport  Port=5
  In6 : Inport  Port=6
  In7 : Inport  Port=7
  In8 : Inport  Port=8
  Demux{1..7} (7 alike) : Demux  Outputs=14
  Multiport Switch{1..7} (7 alike) : MultiPortSwitch  Inputs=13  DataPortForDefault=Additional data port
  Out7 : Outport  VectorParamsAs1DForOutWhenUnconnected=off
  Out1 : Outport  Port=2  VectorParamsAs1DForOutWhenUnconnected=off
  Out2 : Outport  Port=3  VectorParamsAs1DForOutWhenUnconnected=off
  Out3 : Outport  Port=4  VectorParamsAs1DForOutWhenUnconnected=off
  Out4 : Outport  Port=5  VectorParamsAs1DForOutWhenUnconnected=off
  Out5 : Outport  Port=6  VectorParamsAs1DForOutWhenUnconnected=off
  Out6 : Outport  Port=7  VectorParamsAs1DForOutWhenUnconnected=off
  wires:
  In1/1 -> Demux7/1, Demux5/1, Demux4/1, Demux3/1, Demux2/1, Demux1/1, Demux6/1
  In2/1 -> Multiport Switch1/1
  Demux6/9 -> Multiport Switch1/10
  Demux6/8 -> Multiport Switch1/9
  Demux6/7 -> Multiport Switch1/8
  Demux6/6 -> Multiport Switch1/7
  Demux6/4 -> Multiport Switch1/5
  Demux6/5 -> Multiport Switch1/6
  Demux6/3 -> Multiport Switch1/4
  Demux6/2 -> Multiport Switch1/3
  Demux6/1 -> Multiport Switch1/2
  Multiport Switch1/1 -> Out7/1
  Demux6/10 -> Multiport Switch1/11
  Demux6/11 -> Multiport Switch1/12
  Demux6/13 -> Multiport Switch1/14
  Demux6/14 -> Multiport Switch1/15
  Demux6/12 -> Multiport Switch1/13
  Demux1/12 -> Multiport Switch2/13
  Demux1/14 -> Multiport Switch2/15
  Demux1/13 -> Multiport Switch2/14
  Demux1/11 -> Multiport Switch2/12
  Demux1/10 -> Multiport Switch2/11
  Multiport Switch2/1 -> Out1/1
  Demux1/1 -> Multiport Switch2/2
  Demux1/2 -> Multiport Switch2/3
  Demux1/3 -> Multiport Switch2/4
  Demux1/5 -> Multiport Switch2/6
  Demux1/4 -> Multiport Switch2/5
  Demux1/6 -> Multiport Switch2/7
  Demux1/7 -> Multiport Switch2/8
  Demux1/8 -> Multiport Switch2/9
  Demux1/9 -> Multiport Switch2/10
  In3/1 -> Multiport Switch2/1
  In4/1 -> Multiport Switch3/1
  Demux2/9 -> Multiport Switch3/10
  Demux2/8 -> Multiport Switch3/9
  Demux2/7 -> Multiport Switch3/8
  Demux2/6 -> Multiport Switch3/7
  Demux2/4 -> Multiport Switch3/5
  Demux2/5 -> Multiport Switch3/6
  Demux2/3 -> Multiport Switch3/4
  Demux2/2 -> Multiport Switch3/3
  Demux2/1 -> Multiport Switch3/2
  Multiport Switch3/1 -> Out2/1
  Demux2/10 -> Multiport Switch3/11
  Demux2/11 -> Multiport Switch3/12
  Demux2/13 -> Multiport Switch3/14
  Demux2/14 -> Multiport Switch3/15
  Demux2/12 -> Multiport Switch3/13
  Demux3/12 -> Multiport Switch4/13
  Demux3/14 -> Multiport Switch4/15
  Demux3/13 -> Multiport Switch4/14
  Demux3/11 -> Multiport Switch4/12
  Demux3/10 -> Multiport Switch4/11
  Multiport Switch4/1 -> Out3/1
  Demux3/1 -> Multiport Switch4/2
  Demux3/2 -> Multiport Switch4/3
  Demux3/3 -> Multiport Switch4/4
  Demux3/5 -> Multiport Switch4/6
  Demux3/4 -> Multiport Switch4/5
  Demux3/6 -> Multiport Switch4/7
  Demux3/7 -> Multiport Switch4/8
  Demux3/8 -> Multiport Switch4/9
  Demux3/9 -> Multiport Switch4/10
  In5/1 -> Multiport Switch4/1
  In6/1 -> Multiport Switch5/1
  Demux4/9 -> Multiport Switch5/10
  Demux4/8 -> Multiport Switch5/9
  Demux4/7 -> Multiport Switch5/8
  Demux4/6 -> Multiport Switch5/7
  Demux4/4 -> Multiport Switch5/5
  Demux4/5 -> Multiport Switch5/6
  Demux4/3 -> Multiport Switch5/4
  Demux4/2 -> Multiport Switch5/3
  Demux4/1 -> Multiport Switch5/2
  Multiport Switch5/1 -> Out4/1
  Demux4/10 -> Multiport Switch5/11
  Demux4/11 -> Multiport Switch5/12
  Demux4/13 -> Multiport Switch5/14
  Demux4/14 -> Multiport Switch5/15
  Demux4/12 -> Multiport Switch5/13
  Demux5/12 -> Multiport Switch6/13
  Demux5/14 -> Multiport Switch6/15
  Demux5/13 -> Multiport Switch6/14
  Demux5/11 -> Multiport Switch6/12
  Demux5/10 -> Multiport Switch6/11
  Multiport Switch6/1 -> Out5/1
  Demux5/1 -> Multiport Switch6/2
  Demux5/2 -> Multiport Switch6/3
  Demux5/3 -> Multiport Switch6/4
  Demux5/5 -> Multiport Switch6/6
  Demux5/4 -> Multiport Switch6/5
  Demux5/6 -> Multiport Switch6/7
  Demux5/7 -> Multiport Switch6/8
  Demux5/8 -> Multiport Switch6/9
  Demux5/9 -> Multiport Switch6/10
  In7/1 -> Multiport Switch6/1
  In8/1 -> Multiport Switch7/1
  Demux7/9 -> Multiport Switch7/10
  Demux7/8 -> Multiport Switch7/9
  Demux7/7 -> Multiport Switch7/8
  Demux7/6 -> Multiport Switch7/7
  Demux7/4 -> Multiport Switch7/5
  Demux7/5 -> Multiport Switch7/6
  Demux7/3 -> Multiport Switch7/4
  Demux7/2 -> Multiport Switch7/3
  Demux7/1 -> Multiport Switch7/2
  Multiport Switch7/1 -> Out6/1
  Demux7/10 -> Multiport Switch7/11
  Demux7/11 -> Multiport Switch7/12
  Demux7/13 -> Multiport Switch7/14
  Demux7/14 -> Multiport Switch7/15
  Demux7/12 -> Multiport Switch7/13

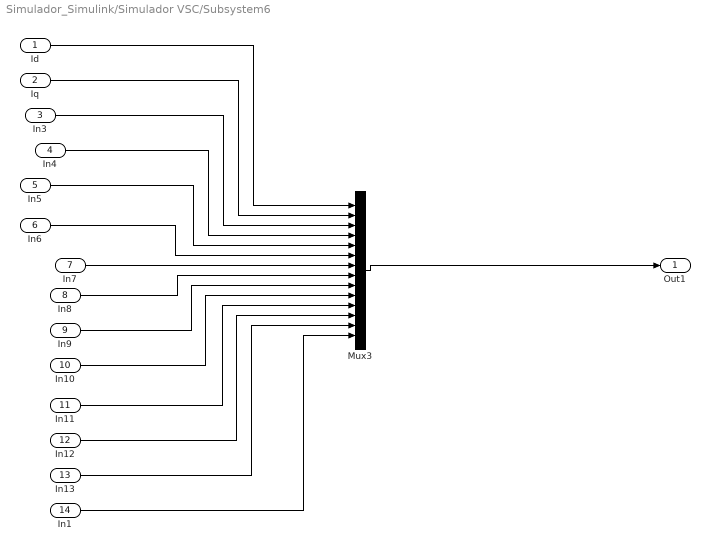
== system Simulador_Simulink/Simulador VSC/Subsystem6 ==
  Id : Inport
  Iq : Inport  Port=2
  In3 : Inport  Port=3
  In4 : Inport  Port=4
  In5 : Inport  Port=5
  In6 : Inport  Port=6
  In7 : Inport  Port=7
  In8 : Inport  Port=8
  In9 : Inport  Port=9
  In10 : Inport  Port=10
  In11 : Inport  Port=11
  In12 : Inport  Port=12
  In13 : Inport  Port=13
  In1 : Inport  Port=14
  Mux3 : Mux  Inputs=14
  Out1 : Outport  VectorParamsAs1DForOutWhenUnconnected=off
  wires:
  Mux3/1 -> Out1/1
  In7/1 -> Mux3/7
  Iq/1 -> Mux3/2
  In5/1 -> Mux3/5
  In12/1 -> Mux3/12
  In9/1 -> Mux3/9
  In10/1 -> Mux3/10
  In3/1 -> Mux3/3
  In6/1 -> Mux3/6
  In4/1 -> Mux3/4
  Id/1 -> Mux3/1
  In13/1 -> Mux3/13
  In8/1 -> Mux3/8
  In11/1 -> Mux3/11
  In1/1 -> Mux3/14

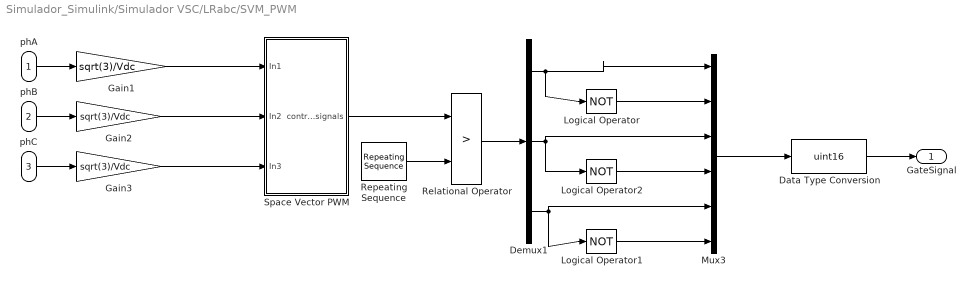
== system Simulador_Simulink/Simulador VSC/LRabc/SVM_PWM ==
  phA : Inport
  phB : Inport  Port=2
  phC : Inport  Port=3
  Data Type Conversion : DataTypeConversion  OutDataTypeStr=uint16
  Demux1 : Demux  Outputs=3
  Gain1 : Gain  Gain=sqrt(3)/Vdc
  Gain2 : Gain  Gain=sqrt(3)/Vdc
  Gain3 : Gain  Gain=sqrt(3)/Vdc
  Logical Operator : Logic  Operator=NOT  AllPortsSameDT=off  OutDataTypeStr=boolean
  Logical Operator1 : Logic  Operator=NOT  AllPortsSameDT=off  OutDataTypeStr=boolean
  Logical Operator2 : Logic  Operator=NOT  AllPortsSameDT=off  OutDataTypeStr=boolean
  Mux3 : Mux  Inputs=6
  Relational Operator : RelationalOperator  Operator=>  RndMeth=Nearest
  Repeating Sequence : simulink/Sources/Repeating Sequence  rep_seq_t=[0 0.25/Freq_Conmutacion 0.5/Freq_Conmutacion 0.75/Freq_Conmutacion 1/Freq_Conmutacion]  rep_seq_y=[1 0 -1 0 1]
  Space Vector PWM : Subsystem
  GateSignal : Outport  VectorParamsAs1DForOutWhenUnconnected=off
  wires:
  phA/1 -> Gain1/1
  phB/1 -> Gain2/1
  phC/1 -> Gain3/1
  Mux3/1 -> Data Type Conversion/1
  Gain2/1 -> Space Vector PWM/2(In2)
  Gain3/1 -> Space Vector PWM/3(In3)
  Gain1/1 -> Space Vector PWM/1(In1)
  Logical Operator/1 -> Mux3/2
  Demux1/1 -> Logical Operator/1, Mux3/1
  Logical Operator2/1 -> Mux3/4
  Logical Operator1/1 -> Mux3/6
  Relational Operator/1 -> Demux1/1
  Demux1/2 -> Logical Operator2/1, Mux3/3
  Demux1/3 -> Logical Operator1/1, Mux3/5
  Space Vector PWM/1(control_signals) -> Relational Operator/1
  Data Type Conversion/1 -> GateSignal/1
  Repeating Sequence/1 -> Relational Operator/2

== system Simulador_Simulink/Simulador VSC/Subsystem/Control P fase d ==
  In1 : Inport
  In2 : Inport  Port=2
  Gain10 : Gain  Gain=Control_P
  Gain6 : Gain  Gain=K_proporcional
  Sum2 : Sum  Inputs=|+-
  Out1 : Outport  VectorParamsAs1DForOutWhenUnconnected=off
  wires:
  In1/1 -> Sum2/1
  Gain10/1 -> Out1/1
  In2/1 -> Gain6/1
  Sum2/1 -> Gain10/1
  Gain6/1 -> Sum2/2

== system Simulador_Simulink/Simulador VSC/Subsystem/Control P fase q ==
  In1 : Inport
  In2 : Inport  Port=2
  Gain7 : Gain  Gain=K_proporcional
  Gain9 : Gain  Gain=Control_P
  Sum4 : Sum  Inputs=|+-
  Out1 : Outport  VectorParamsAs1DForOutWhenUnconnected=off
  wires:
  Gain9/1 -> Out1/1
  In2/1 -> Gain7/1
  Sum4/1 -> Gain9/1
  In1/1 -> Sum4/1
  Gain7/1 -> Sum4/2

== system Simulador_Simulink/Simulador VSC/Subsystem4/Salidas No Reales Simuladas ==
  PWM1A : Inport
  PWM1B : Inport  Port=2
  PWM2A : Inport  Port=3
  PWM2B : Inport  Port=4
  PWM3A : Inport  Port=5
  PWM3B : Inport  Port=6
  DAC-A : Inport  Port=7
  "Salidas Selecionadas Medidas " : Scope  NumInputPorts=7
  wires:
  PWM3A/1 -> "Salidas Selecionadas Medidas "/5  "PWM3A"
  PWM1A/1 -> "Salidas Selecionadas Medidas "/1  "PWM1A"
  PWM3B/1 -> "Salidas Selecionadas Medidas "/6  "PWM3B"
  PWM1B/1 -> "Salidas Selecionadas Medidas "/2  "PWM1B"
  DAC-A/1 -> "Salidas Selecionadas Medidas "/7  "DAC-A"
  PWM2A/1 -> "Salidas Selecionadas Medidas "/3  "PWM2A"
  PWM2B/1 -> "Salidas Selecionadas Medidas "/4  "PWM2B"

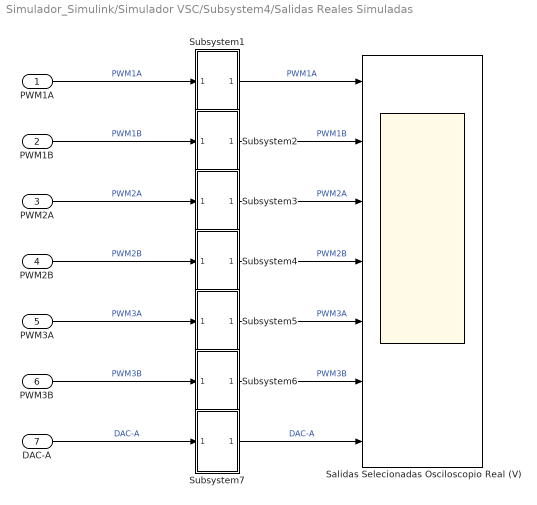
== system Simulador_Simulink/Simulador VSC/Subsystem4/Salidas Reales Simuladas ==
  PWM1A : Inport
  PWM1B : Inport  Port=2
  PWM2A : Inport  Port=3
  PWM2B : Inport  Port=4
  PWM3A : Inport  Port=5
  PWM3B : Inport  Port=6
  DAC-A : Inport  Port=7
  Salidas Selecionadas Osciloscopio Real (V) : Scope  NumInputPorts=7
  Subsystem1 : Subsystem
  Subsystem2 : Subsystem
  Subsystem3 : Subsystem
  Subsystem4 : Subsystem
  Subsystem5 : Subsystem
  Subsystem6 : Subsystem
  Subsystem7 : Subsystem
  wires:
  PWM2B/1 -> Subsystem4/1(In1)  "PWM2B"
  PWM2A/1 -> Subsystem3/1(In1)  "PWM2A"
  DAC-A/1 -> Subsystem7/1(In1)  "DAC-A"
  PWM1B/1 -> Subsystem2/1(In1)  "PWM1B"
  PWM3B/1 -> Subsystem6/1(In1)  "PWM3B"
  PWM1A/1 -> Subsystem1/1(In1)  "PWM1A"
  PWM3A/1 -> Subsystem5/1(In1)  "PWM3A"
  Subsystem1/1(Out1) -> Salidas Selecionadas Osciloscopio Real (V)/1  "PWM1A"
  Subsystem2/1(Out1) -> Salidas Selecionadas Osciloscopio Real (V)/2  "PWM1B"
  Subsystem3/1(Out1) -> Salidas Selecionadas Osciloscopio Real (V)/3  "PWM2A"
  Subsystem4/1(Out1) -> Salidas Selecionadas Osciloscopio Real (V)/4  "PWM2B"
  Subsystem5/1(Out1) -> Salidas Selecionadas Osciloscopio Real (V)/5  "PWM3A"
  Subsystem6/1(Out1) -> Salidas Selecionadas Osciloscopio Real (V)/6  "PWM3B"
  Subsystem7/1(Out1) -> Salidas Selecionadas Osciloscopio Real (V)/7  "DAC-A"

== system Simulador_Simulink/Simulador VSC/LRabc/SVM_PWM/Space Vector PWM ==
  In1 : Inport
  In2 : Inport  Port=2
  In3 : Inport  Port=3
  Gain1 : Gain  Gain=2/sqrt(3)
  Mux3 : Mux  Inputs=3
  modulation index2 : Gain  Gain=m  SaturateOnIntegerOverflow=on  OutDataTypeStr=Inherit: Same as input  ParamDataTypeStr=Inherit: Same as input
  control_signals : Outport  VectorParamsAs1DForOutWhenUnconnected=off
  wires:
  Mux3/1 -> modulation index2/1
  modulation index2/1 -> Gain1/1
  Gain1/1 -> control_signals/1
  In3/1 -> Mux3/3
  In2/1 -> Mux3/2
  In1/1 -> Mux3/1

== system Simulador_Simulink/Simulador VSC/Subsystem4/Salidas Reales Simuladas/Subsystem1 ==
  In1 : Inport
  Constant : Constant  Value=1.5
  Gain : Gain  Gain=0.5
  Gain2 : Gain  Gain=1.5
  Sum : Sum  Inputs=|++
  Out1 : Outport  VectorParamsAs1DForOutWhenUnconnected=off
  wires:
  Constant/1 -> Sum/2
  Sum/1 -> Out1/1
  Gain2/1 -> Sum/1
  In1/1 -> Gain/1
  Gain/1 -> Gain2/1

== system Simulador_Simulink/Simulador VSC/Subsystem4/Salidas Reales Simuladas/Subsystem2 ==
  In1 : Inport
  Constant : Constant  Value=1.5
  Gain : Gain  Gain=0.5
  Gain2 : Gain  Gain=1.5
  Sum : Sum  Inputs=|++
  Out1 : Outport  VectorParamsAs1DForOutWhenUnconnected=off
  wires:
  Gain/1 -> Gain2/1
  In1/1 -> Gain/1
  Gain2/1 -> Sum/1
  Sum/1 -> Out1/1
  Constant/1 -> Sum/2

== system Simulador_Simulink/Simulador VSC/Subsystem4/Salidas Reales Simuladas/Subsystem3 ==
  In1 : Inport
  Constant : Constant  Value=1.5
  Gain : Gain  Gain=0.5
  Gain2 : Gain  Gain=1.5
  Sum : Sum  Inputs=|++
  Out1 : Outport  VectorParamsAs1DForOutWhenUnconnected=off
  wires:
  Constant/1 -> Sum/2
  Sum/1 -> Out1/1
  Gain2/1 -> Sum/1
  In1/1 -> Gain/1
  Gain/1 -> Gain2/1

== system Simulador_Simulink/Simulador VSC/Subsystem4/Salidas Reales Simuladas/Subsystem4 ==
  In1 : Inport
  Constant : Constant  Value=1.5
  Gain : Gain  Gain=0.5
  Gain2 : Gain  Gain=1.5
  Sum : Sum  Inputs=|++
  Out1 : Outport  VectorParamsAs1DForOutWhenUnconnected=off
  wires:
  Gain/1 -> Gain2/1
  In1/1 -> Gain/1
  Gain2/1 -> Sum/1
  Sum/1 -> Out1/1
  Constant/1 -> Sum/2

== system Simulador_Simulink/Simulador VSC/Subsystem4/Salidas Reales Simuladas/Subsystem5 ==
  In1 : Inport
  Constant : Constant  Value=1.5
  Gain : Gain  Gain=3.3
  Gain2 : Gain  Gain=1/80
  Sum : Sum  Inputs=|++
  Out1 : Outport  VectorParamsAs1DForOutWhenUnconnected=off
  wires:
  Constant/1 -> Sum/2
  Sum/1 -> Out1/1
  In1/1 -> Gain2/1
  Gain2/1 -> Gain/1
  Gain/1 -> Sum/1

== system Simulador_Simulink/Simulador VSC/Subsystem4/Salidas Reales Simuladas/Subsystem6 ==
  In1 : Inport
  Constant : Constant  Value=1.5
  Gain2 : Gain  Gain=0.1
  Sum : Sum  Inputs=|++
  Out1 : Outport  VectorParamsAs1DForOutWhenUnconnected=off
  wires:
  In1/1 -> Gain2/1
  Sum/1 -> Out1/1
  Constant/1 -> Sum/2
  Gain2/1 -> Sum/1

== system Simulador_Simulink/Simulador VSC/Subsystem4/Salidas Reales Simuladas/Subsystem7 ==
  In1 : Inport
  Constant : Constant  Value=1.5
  Gain : Gain  Gain=0.2
  Sum : Sum  Inputs=|++
  Out1 : Outport  VectorParamsAs1DForOutWhenUnconnected=off
  wires:
  Constant/1 -> Sum/2
  Sum/1 -> Out1/1
  Gain/1 -> Sum/1
  In1/1 -> Gain/1
